simulink model "rocket_thrust_data_test_model"  (R2014a)
settings: Solver=ode45  StartTime=0.0  StopTime=10.0  RelTol=1e-3
libraries: rocket_thrust_data_library x1, rocket_dynamic_data_library x1
settings Model: Creator=scorpii  LastModifiedBy=scorpii

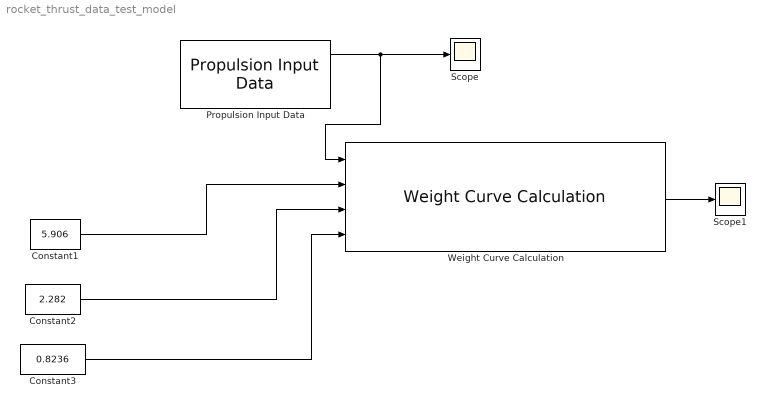
== system rocket_thrust_data_test_model ==
  Constant1 : Constant  Value=5.906
  Constant2 : Constant  Value=2.282
  Constant3 : Constant  Value=0.8236
  Propulsion Input Data : rocket_thrust_data_library/Propulsion Input Data
  Scope : Scope
  Scope1 : Scope
  Weight Curve Calculation : rocket_dynamic_data_library/Weight Curve Calculation
  wires:
  Propulsion Input Data/1 -> Weight Curve Calculation/1, Scope/1
  Constant1/1 -> Weight Curve Calculation/2
  Constant2/1 -> Weight Curve Calculation/3
  Constant3/1 -> Weight Curve Calculation/4
  Weight Curve Calculation/1 -> Scope1/1
